simulink model "MLCSI_2"  (R2024a)
settings: Solver=FixedStepAuto  StartTime=0.0  StopTime=0.3  FixedStep=1e-6  RelTol=1e-3
undefined symbols (not defined in the file): Am, Cf, L, LL, RL
libraries: spsCurrentMeasurementLib x12, spsDiodeLib x12, spsIGBTDiodeLib x12, spsSeriesRLCBranchLib x11, spsVoltageMeasurementLib x8, spsIdealSwitchLib x2, spsControlledCurrentSourceLib x1, spsGroundLib x1, spspowerguiLib x1
(part 1 of 2)
settings Model: Creator=Muyu Chen  LastModifiedBy=muyu
settings DataIOCC: ReturnWorkspaceOutputs=off
settings DebuggingCC: UnconnectedInputMsg=warning  UnconnectedOutputMsg=warning  UnconnectedLineMsg=warning
settings ModelReferenceCC: EnableRefExpFcnMdlSchedulingChecks=on
settings RTWCC: GPUComputeCapability=3.5  DLArmComputeVersion=19.05

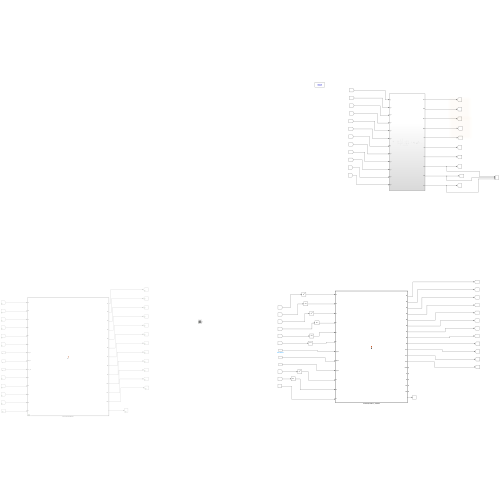
[thumbnail: Simulink's stored preview of the top-level diagram]
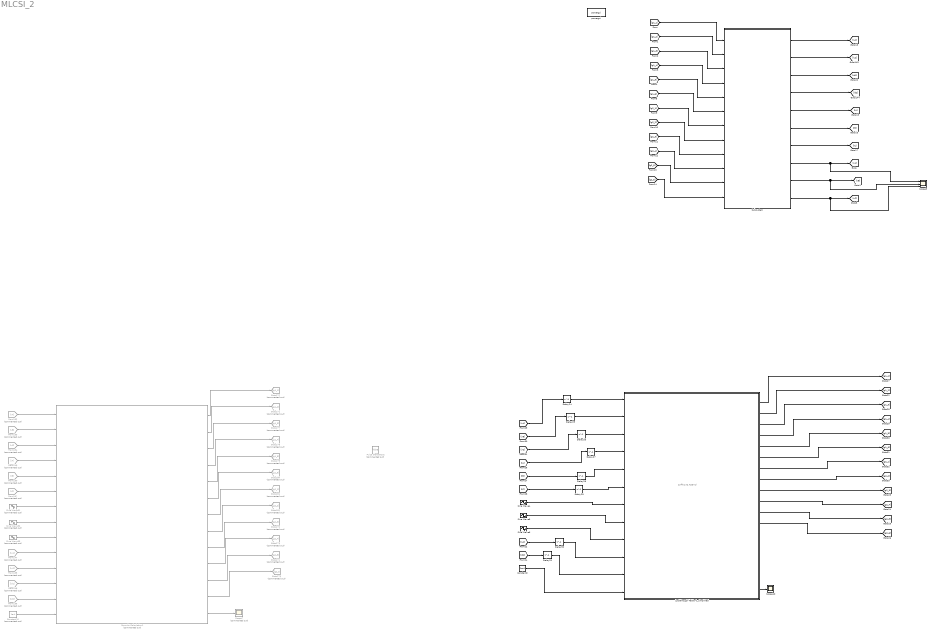
== system MLCSI_2 ==
  note: surf(K1,K2,K2DV1)
  Constant16 : Constant  Commented=on  Value=1e-4
  Constant2 : Constant  Value=1e-4
  Delay{24..31} (8 alike) : Delay  DelayLength=1  InitialCondition=0
  Formula Calculation1 : MATLAB Function  Commented=on  TreatAsAtomicUnit=on
  From147 : From  Commented=on  GotoTag=iu1
  From148 : From  Commented=on  GotoTag=id1
  From149 : From  Commented=on  GotoTag=iA
  From150 : From  Commented=on  GotoTag=iB
  From151 : From  Commented=on  GotoTag=iC
  From152 : From  Commented=on  GotoTag=vA
  From153 : From  Commented=on  GotoTag=vB
  From154 : From  Commented=on  GotoTag=vC
  From155 : From  Commented=on  GotoTag=iu2
  From156 : From  Commented=on  GotoTag=id2
  Goto171 : Goto  Commented=on  GotoTag=g1_2
  Goto172 : Goto  Commented=on  GotoTag=g2_3
  Goto173 : Goto  Commented=on  GotoTag=g2_4
  Goto174 : Goto  Commented=on  GotoTag=g2_5
  Goto175 : Goto  Commented=on  GotoTag=g2_6
  Goto176 : Goto  Commented=on  GotoTag=g1_1
  Goto177 : Goto  Commented=on  GotoTag=g1_3
  Goto178 : Goto  Commented=on  GotoTag=g1_4
  Goto179 : Goto  Commented=on  GotoTag=g1_5
  Goto180 : Goto  Commented=on  GotoTag=g1_6
  Goto181 : Goto  Commented=on  GotoTag=g2_1
  Goto182 : Goto  Commented=on  GotoTag=g2_2
  Lookthrough Table 4_ simplified : MATLAB Function  TreatAsAtomicUnit=on
  Pulse Generator2 : DiscretePulseGenerator  Commented=on  PulseType=Time based  Period=1e-4  PulseWidth=50
  Scope10 : Scope
  Scope5 : Scope  NumInputPorts=3
  Scope7 : Scope  Commented=on
  Sine Wave31 : Sin  Commented=on  Amplitude=Am  Frequency=2*pi*50  SampleTime=1e-6
  Sine Wave32 : Sin  Commented=on  Amplitude=Am  Frequency=2*pi*50  Phase=2*pi/3  SampleTime=1e-6
  Sine Wave33 : Sin  Commented=on  Amplitude=Am  Frequency=2*pi*50  Phase=4*pi/3  SampleTime=1e-6
  Sine Wave4 : Sin  Amplitude=Am  Frequency=2*pi*50  SampleTime=1e-6
  Sine Wave5 : Sin  Amplitude=Am  Frequency=2*pi*50  Phase=2*pi/3  SampleTime=1e-6
  Sine Wave6 : Sin  Amplitude=Am  Frequency=2*pi*50  Phase=4*pi/3  SampleTime=1e-6
  Subsystem : Subsystem
  powergui : spspowerguiLib/powergui  Priority=1  SimulationMode=Discrete  SampleTime=1e-6  frequency=60  Iterations=50  frequencyindice=0  Pbase=100e6  ErrMax=1e-4  UnitsV=kV  UnitsW=MW  buscounter=0  FunctionMessages=off  echomessages=off  EnableUseOfTLC=off  CurrentSourceSwitches=off  DisableSnubberDevices=off  DisableRonSwitches=off  DisableVfSwitches=off  DisplayEquations=off  AutomaticDiscreteSolvers=off  SolverType=Tustin/Backward Euler (TBE)  Interpol=off  ExternalGateDelay=off  methode=off  Ts=100  x0status=blocks  SPID=on  SwTol=0  HookPort=off  NonlinearTolerance=1e-4  nMaxIteration=100  ContinueOnMaxIteration=off  RestoreLinks=warning  ResistiveCurrentMeasurement=off  Frange=[0:2:500]  Ylog=off  Xlog=on  ShowGrid=off  save=off  variable=ZData  structure=0  ZoomFFT=off  StartTime=0.0  cycles=1  DisplayStyle=1  fundamental=60  FreqAxis=off  MaxFrequency=1000  frequencyindicesteady=1  RmsSteady=1  display=off
  wires:
  [g1_5] -> Subsystem/5(1_5)
  Subsystem/3(id1) -> [id1]
  Subsystem/7(ic) -> [iC]
  [g1_4] -> Subsystem/4(1_4)
  Subsystem/9(ub) -> Scope5/2, [vB]
  [g2_2] -> Subsystem/8(2_2)
  Subsystem/4(id2) -> [id2]
  Subsystem/5(ia) -> [iA]
  Subsystem/6(ib) -> [iB]
  [g2_3] -> Subsystem/9(2_3)
  [g1_2] -> Subsystem/2(1_2)
  Subsystem/1(iu1) -> [iu1]
  Subsystem/8(ua) -> Scope5/1, [vA]
  [g2_4] -> Subsystem/10(2_4)
  [g1_6] -> Subsystem/6(1_6)
  [g2_1] -> Subsystem/7(2_1)
  Subsystem/10(uc) -> [vC], Scope5/3
  Subsystem/2(iu2) -> [iu2]
  [g2_5] -> Subsystem/11(2_5)
  [g2_6] -> Subsystem/12(2_6)
  [g1_3] -> Subsystem/3(1_3)
  [g1_1] -> Subsystem/1(1_1)
  Sine Wave5/1 -> Lookthrough Table 4_ simplified/8(vB_ref)
  [vA] -> Delay24/1
  [vB] -> Delay25/1
  [vC] -> Delay26/1
  [iA] -> Delay27/1
  [iB] -> Delay28/1
  [iC] -> Delay29/1
  Sine Wave4/1 -> Lookthrough Table 4_ simplified/7(vA_ref)
  Sine Wave6/1 -> Lookthrough Table 4_ simplified/9(vC_ref)
  [iu1] -> Delay30/1
  [id1] -> Delay31/1
  Constant2/1 -> Lookthrough Table 4_ simplified/12(Ts)
  Lookthrough Table 4_ simplified/1(S1) -> [g1_1]
  Lookthrough Table 4_ simplified/2(S2) -> [g1_2]
  Lookthrough Table 4_ simplified/3(S3) -> [g1_3]
  Lookthrough Table 4_ simplified/4(S4) -> [g1_4]
  Lookthrough Table 4_ simplified/5(S5) -> [g1_5]
  Lookthrough Table 4_ simplified/6(S6) -> [g1_6]
  Lookthrough Table 4_ simplified/7(S7) -> [g2_1]
  Lookthrough Table 4_ simplified/8(S8) -> [g2_2]
  Lookthrough Table 4_ simplified/9(S9) -> [g2_3]
  Lookthrough Table 4_ simplified/10(S10) -> [g2_4]
  Lookthrough Table 4_ simplified/11(S11) -> [g2_5]
  Lookthrough Table 4_ simplified/12(S12) -> [g2_6]
  Formula Calculation1/11(S11) -> Goto174/1
  From147/1 -> Formula Calculation1/10(iu1)
  From149/1 -> Formula Calculation1/4(iA)
  Formula Calculation1/7(S7) -> Goto181/1
  Formula Calculation1/6(S6) -> Goto180/1
  Sine Wave32/1 -> Formula Calculation1/8(vB_ref)
  Sine Wave31/1 -> Formula Calculation1/7(vA_ref)
  From154/1 -> Formula Calculation1/3(vC)
  Formula Calculation1/3(S3) -> Goto177/1
  From156/1 -> Formula Calculation1/13(id2)
  Formula Calculation1/4(S4) -> Goto178/1
  Formula Calculation1/8(S8) -> Goto182/1
  From150/1 -> Formula Calculation1/5(iB)
  Formula Calculation1/9(S9) -> Goto172/1
  From153/1 -> Formula Calculation1/2(vB)
  Formula Calculation1/5(S5) -> Goto179/1
  Formula Calculation1/2(S2) -> Goto171/1
  Formula Calculation1/13(t) -> Scope7/1
  Formula Calculation1/1(S1) -> Goto176/1
  From148/1 -> Formula Calculation1/12(id1)
  From155/1 -> Formula Calculation1/11(iu2)
  From151/1 -> Formula Calculation1/6(iC)
  From152/1 -> Formula Calculation1/1(vA)
  Constant16/1 -> Formula Calculation1/14(Ts)
  Formula Calculation1/12(S12) -> Goto175/1
  Formula Calculation1/10(S10) -> Goto173/1
  Sine Wave33/1 -> Formula Calculation1/9(vC_ref)
  Delay24/1 -> Lookthrough Table 4_ simplified/1(va)
  Delay25/1 -> Lookthrough Table 4_ simplified/2(vb)
  Delay26/1 -> Lookthrough Table 4_ simplified/3(vc)
  Delay27/1 -> Lookthrough Table 4_ simplified/4(iA)
  Delay28/1 -> Lookthrough Table 4_ simplified/5(iB)
  Delay29/1 -> Lookthrough Table 4_ simplified/6(iC)
  Delay30/1 -> Lookthrough Table 4_ simplified/10(iu1)
  Delay31/1 -> Lookthrough Table 4_ simplified/11(id1)
  Lookthrough Table 4_ simplified/18(t) -> Scope10/1

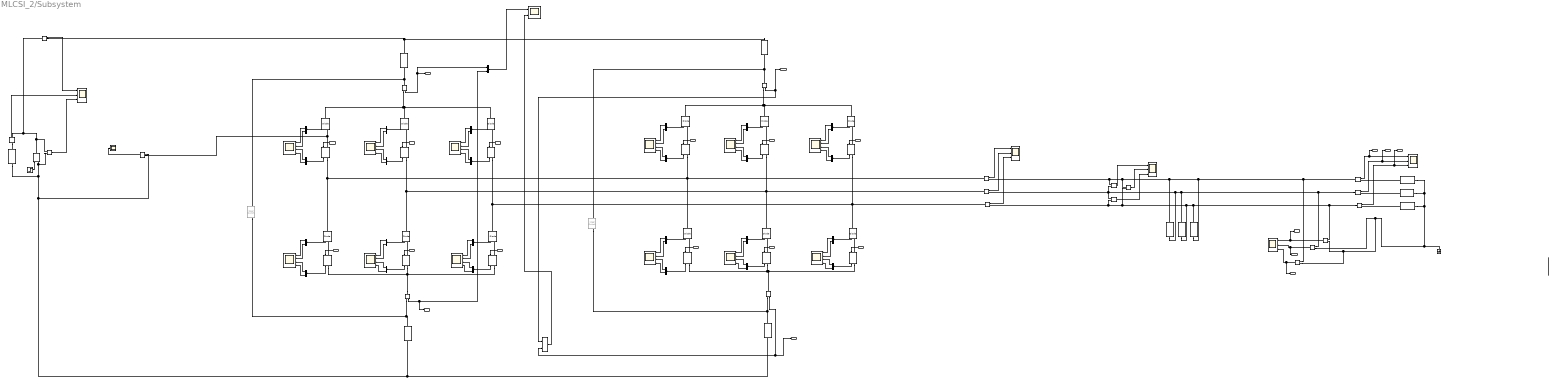
== system MLCSI_2/Subsystem ==
  1_1 : Inport
  1_2 : Inport  Port=2
  1_3 : Inport  Port=3
  1_4 : Inport  Port=4
  1_5 : Inport  Port=5
  1_6 : Inport  Port=6
  2_1 : Inport  Port=7
  2_2 : Inport  Port=8
  2_3 : Inport  Port=9
  2_4 : Inport  Port=10
  2_5 : Inport  Port=11
  2_6 : Inport  Port=12
  Controlled Current Source : spsControlledCurrentSourceLib/Controlled Current Source  Initialize=on  Source_Type=DC  Amplitude=0  Phase=0  Frequency=0  Measurements=None
  Current Measurement{,1..11} (12 alike) : spsCurrentMeasurementLib/Current Measurement  PhasorSimulation=off  OutputType=Complex  PSBequivalent=0
  Demux{,1..23} (24 alike) : Demux  Outputs=2
  Diode{,1..11} (12 alike) : spsDiodeLib/Diode  Ron=1e-3  Lon=0  Vf=0  IC=0  UseSnubber=0  Rs=1e6  Cs=inf  Measurements=on
  Ground : spsGroundLib/Ground  LConnTagsString=a
  IGBT/Diode{,1..11} (12 alike) : spsIGBTDiodeLib/IGBT//Diode  Ron=1e-3  Rs=1e5  Cs=inf  Measurements=on
  Ideal Switch : spsIdealSwitchLib/Ideal Switch  Commented=on  Ron=0.0001  Lon=0  IC=1  Rs=inf  Cs=inf  Measurements=on
  Ideal Switch1 : spsIdealSwitchLib/Ideal Switch  Commented=on  Ron=0.0001  Lon=0  IC=1  Rs=inf  Cs=inf  Measurements=on
  Mux : Mux  Inputs=2
  Mux1 : Mux  Inputs=2
  Scope{,1..3,20} (5 alike) : Scope  NumInputPorts=3
  Scope{5..10,12,15..19} (12 alike) : Scope  NumInputPorts=4
  Scope11 : Scope  NumInputPorts=2
  Scope4 : Scope
  Series RLC Branch{1,9..11} (4 alike) : spsSeriesRLCBranchLib/Series RLC Branch  LConnTagsString=__new0  RConnTagsString=__new0  BranchType=L  Resistance=30  Inductance=L  SetiL0=off  InitialCurrent=0  Capacitance=1e-6  Setx0=off  InitialVoltage=0  Measurements=None
  Series RLC Branch2 : spsSeriesRLCBranchLib/Series RLC Branch  LConnTagsString=__new0  RConnTagsString=__new0  BranchType=R  Resistance=1e11  Inductance=165e-3  SetiL0=off  InitialCurrent=0  Capacitance=1e-6  Setx0=off  InitialVoltage=0  Measurements=None
  Series RLC Branch3 : spsSeriesRLCBranchLib/Series RLC Branch  LConnTagsString=__new0  RConnTagsString=__new0  BranchType=RL  Resistance=RL  Inductance=LL  SetiL0=off  InitialCurrent=0  Capacitance=1e-6  Setx0=off  InitialVoltage=0  Measurements=None
  Series RLC Branch4 : spsSeriesRLCBranchLib/Series RLC Branch  LConnTagsString=__new0  RConnTagsString=__new0  BranchType=RL  Resistance=RL  Inductance=LL  SetiL0=off  InitialCurrent=0  Capacitance=1e-6  Setx0=off  InitialVoltage=0  Measurements=None
  Series RLC Branch5 : spsSeriesRLCBranchLib/Series RLC Branch  LConnTagsString=__new0  RConnTagsString=__new0  BranchType=RL  Resistance=RL  Inductance=LL  SetiL0=off  InitialCurrent=0  Capacitance=1e-6  Setx0=off  InitialVoltage=0  Measurements=None
  Series RLC Branch6 : spsSeriesRLCBranchLib/Series RLC Branch  LConnTagsString=__new0  RConnTagsString=__new0  BranchType=C  Resistance=30  Inductance=165e-3  SetiL0=off  InitialCurrent=0  Capacitance=Cf  Setx0=off  InitialVoltage=0  Measurements=None
  Series RLC Branch7 : spsSeriesRLCBranchLib/Series RLC Branch  LConnTagsString=__new0  RConnTagsString=__new0  BranchType=C  Resistance=30  Inductance=165e-3  SetiL0=off  InitialCurrent=0  Capacitance=Cf  Setx0=off  InitialVoltage=0  Measurements=None
  Series RLC Branch8 : spsSeriesRLCBranchLib/Series RLC Branch  LConnTagsString=__new0  RConnTagsString=__new0  BranchType=C  Resistance=30  Inductance=165e-3  SetiL0=off  InitialCurrent=0  Capacitance=Cf  Setx0=off  InitialVoltage=0  Measurements=None
  Step : Step  Time=0  After=100  SampleTime=0
  Voltage Measurement{,1,3..8} (8 alike) : spsVoltageMeasurementLib/Voltage Measurement  PhasorSimulation=off  OutputType=Complex  PSBequivalent=0
  iu1 : Outport
  iu2 : Outport  Port=2
  id1 : Outport  Port=3
  id2 : Outport  Port=4
  ia : Outport  Port=5
  ib : Outport  Port=6
  ic : Outport  Port=7
  ua : Outport  Port=8
  ub : Outport  Port=9
  uc : Outport  Port=10
  wires:
  Step/1 -> Controlled Current Source/1
  1_1/1 -> IGBT/Diode/1
  1_2/1 -> IGBT/Diode1/1
  1_3/1 -> IGBT/Diode2/1
  1_4/1 -> IGBT/Diode3/1
  1_5/1 -> IGBT/Diode4/1
  1_6/1 -> IGBT/Diode5/1
  Voltage Measurement6/1 -> Scope1/1  "vab"
  Voltage Measurement8/1 -> Scope1/2  "vac"
  Voltage Measurement7/1 -> Scope1/3  "vbc"
  Current Measurement4/1 -> Scope2/1  "i_inva"
  Current Measurement5/1 -> Scope2/2  "i_invb"
  Current Measurement6/1 -> Scope2/3  "i_invc"
  Current Measurement1/1 -> Scope3/1  "Idc"
  Current Measurement/1 -> Scope3/2  "I_short"
  Voltage Measurement/1 -> Scope3/3  "Vsource"
  Current Measurement2/1 -> Mux/1, iu1/1  "I_LU"
  Current Measurement3/1 -> id1/1, Mux/2  "I_LD"
  Diode/1 -> Demux/1
  IGBT/Diode/1 -> Demux1/1
  Demux/1 -> Scope5/1
  Demux/2 -> Scope5/2
  Demux1/1 -> Scope5/3
  Demux1/2 -> Scope5/4
  Demux3/1 -> Scope6/3
  Demux2/1 -> Scope6/1
  IGBT/Diode3/1 -> Demux3/1
  Demux2/2 -> Scope6/2
  Demux3/2 -> Scope6/4
  Diode3/1 -> Demux2/1
  Demux5/1 -> Scope7/3
  Demux4/1 -> Scope7/1
  IGBT/Diode1/1 -> Demux5/1
  Demux4/2 -> Scope7/2
  Demux5/2 -> Scope7/4
  Diode1/1 -> Demux4/1
  Demux7/1 -> Scope8/3
  Demux6/1 -> Scope8/1
  IGBT/Diode2/1 -> Demux7/1
  Demux6/2 -> Scope8/2
  Demux7/2 -> Scope8/4
  Diode2/1 -> Demux6/1
  Demux9/1 -> Scope9/3
  Demux8/1 -> Scope9/1
  IGBT/Diode4/1 -> Demux9/1
  Demux8/2 -> Scope9/2
  Demux9/2 -> Scope9/4
  Diode4/1 -> Demux8/1
  IGBT/Diode5/1 -> Demux11/1
  Diode5/1 -> Demux10/1
  Demux11/2 -> Scope10/4
  Demux10/1 -> Scope10/1
  Demux10/2 -> Scope10/2
  Demux11/1 -> Scope10/3
  Diode11/1 -> Demux14/1
  Demux15/2 -> Scope12/4
  Demux22/2 -> Scope19/2
  Diode6/1 -> Demux12/1
  Demux21/2 -> Scope18/4
  IGBT/Diode8/1 -> Demux21/1
  Demux22/1 -> Scope19/1
  IGBT/Diode9/1 -> Demux17/1
  2_5/1 -> IGBT/Diode10/1
  Demux18/1 -> Scope17/1
  Demux16/1 -> Scope16/1
  Demux20/1 -> Scope18/1
  Demux17/2 -> Scope16/4
  Demux21/1 -> Scope18/3
  Demux14/2 -> Scope12/2
  IGBT/Diode11/1 -> Demux15/1
  Diode10/1 -> Demux22/1
  Diode9/1 -> Demux16/1
  Diode7/1 -> Demux18/1
  IGBT/Diode7/1 -> Demux19/1
  Demux20/2 -> Scope18/2
  Demux13/1 -> Scope15/3
  Demux17/1 -> Scope16/3
  Demux13/2 -> Scope15/4
  Demux12/1 -> Scope15/1
  Demux12/2 -> Scope15/2
  Demux23/2 -> Scope19/4
  IGBT/Diode6/1 -> Demux13/1
  Current Measurement7/1 -> iu2/1, Mux1/1  "I_LU"
  Demux18/2 -> Scope17/2
  2_1/1 -> IGBT/Diode6/1
  Current Measurement8/1 -> Mux1/2, id2/1  "I_LD"
  2_2/1 -> IGBT/Diode7/1
  Demux14/1 -> Scope12/1
  Diode8/1 -> Demux20/1
  Demux23/1 -> Scope19/3
  2_4/1 -> IGBT/Diode9/1
  Demux19/2 -> Scope17/4
  Demux19/1 -> Scope17/3
  2_3/1 -> IGBT/Diode8/1
  Demux15/1 -> Scope12/3
  2_6/1 -> IGBT/Diode11/1
  Demux16/2 -> Scope16/2
  IGBT/Diode10/1 -> Demux23/1
  Current Measurement9/1 -> ia/1, Scope20/1  "i_inva"
  Current Measurement10/1 -> ib/1, Scope20/2  "i_inva"
  Current Measurement11/1 -> ic/1, Scope20/3  "i_inva"
  Mux1/1 -> Scope11/2
  Mux/1 -> Scope11/1
  Voltage Measurement1/1 -> Scope4/1
  ? -> Ideal Switch/1
  ? -> Ideal Switch1/1
  Voltage Measurement5/1 -> ua/1, Scope/3  "va"
  Voltage Measurement4/1 -> ub/1, Scope/2  "vb"
  Voltage Measurement3/1 -> uc/1, Scope/1  "vc"
  connections:
  IGBT/Diode3/LConn1 -- Diode3/RConn1
  IGBT/Diode4/LConn1 -- Diode4/RConn1
  IGBT/Diode5/LConn1 -- Diode5/RConn1
  Current Measurement/LConn1 -- Series RLC Branch2/LConn1
  Current Measurement/RConn1 -- Current Measurement1/LConn1 -- Controlled Current Source/RConn1 -- Voltage Measurement/LConn1
  Current Measurement2/LConn1 -- Ideal Switch/LConn1 -- Series RLC Branch1/RConn1
  IGBT/Diode/LConn1 -- Voltage Measurement1/LConn1 -- Diode/RConn1
  IGBT/Diode1/LConn1 -- Diode1/RConn1
  IGBT/Diode2/LConn1 -- Diode2/RConn1
  Current Measurement2/RConn1 -- Diode2/LConn1 -- Diode1/LConn1 -- Diode/LConn1
  IGBT/Diode6/RConn1 -- Diode9/LConn1 -- Diode3/LConn1 -- IGBT/Diode/RConn1 -- Current Measurement4/LConn1
  IGBT/Diode7/RConn1 -- Diode10/LConn1 -- IGBT/Diode1/RConn1 -- Diode4/LConn1 -- Current Measurement5/LConn1
  IGBT/Diode8/RConn1 -- Diode5/LConn1 -- IGBT/Diode2/RConn1 -- Current Measurement6/LConn1 -- Diode11/LConn1
  Current Measurement3/LConn1 -- IGBT/Diode5/RConn1 -- IGBT/Diode4/RConn1 -- IGBT/Diode3/RConn1
  Current Measurement10/LConn1 -- Series RLC Branch7/LConn1 -- Series RLC Branch6/RConn1 -- Voltage Measurement7/LConn1 -- Voltage Measurement6/LConn2 -- Current Measurement5/RConn1 -- Voltage Measurement4/LConn1
  Current Measurement11/LConn1 -- Voltage Measurement3/LConn1 -- Series RLC Branch8/LConn1 -- Series RLC Branch7/RConn1 -- Current Measurement6/RConn1 -- Voltage Measurement7/LConn2 -- Voltage Measurement8/LConn2
  Ground/LConn1 -- Voltage Measurement4/LConn2 -- Voltage Measurement5/LConn2 -- Voltage Measurement3/LConn2 -- Series RLC Branch5/RConn1 -- Series RLC Branch4/RConn1 -- Series RLC Branch3/RConn1
  IGBT/Diode9/RConn1 -- IGBT/Diode11/RConn1 -- Current Measurement8/LConn1 -- IGBT/Diode10/RConn1
  Diode7/LConn1 -- Current Measurement7/RConn1 -- Diode6/LConn1 -- Diode8/LConn1
  IGBT/Diode6/LConn1 -- Diode6/RConn1
  IGBT/Diode8/LConn1 -- Diode8/RConn1
  IGBT/Diode9/LConn1 -- Diode9/RConn1
  Current Measurement7/LConn1 -- Ideal Switch1/LConn1 -- Series RLC Branch10/RConn1
  IGBT/Diode7/LConn1 -- Diode7/RConn1
  IGBT/Diode11/LConn1 -- Diode11/RConn1
  IGBT/Diode10/LConn1 -- Diode10/RConn1
  Series RLC Branch11/RConn1 -- Series RLC Branch9/RConn1 -- Voltage Measurement/LConn2 -- Controlled Current Source/LConn1 -- Series RLC Branch2/RConn1 -- Voltage Measurement1/LConn2
  Series RLC Branch3/LConn1 -- Current Measurement9/RConn1
  Series RLC Branch4/LConn1 -- Current Measurement10/RConn1
  Series RLC Branch5/LConn1 -- Current Measurement11/RConn1
  Series RLC Branch8/RConn1 -- Series RLC Branch6/LConn1 -- Current Measurement4/RConn1 -- Voltage Measurement6/LConn1 -- Voltage Measurement8/LConn1 -- Voltage Measurement5/LConn1 -- Current Measurement9/LConn1
  Series RLC Branch1/LConn1 -- Current Measurement1/RConn1 -- Series RLC Branch10/LConn1
  Current Measurement3/RConn1 -- Ideal Switch/RConn1 -- Series RLC Branch9/LConn1
  Current Measurement8/RConn1 -- Ideal Switch1/RConn1 -- Series RLC Branch11/LConn1
  ?
